simulink model "submarine"  (Simulink 6.3)
settings: Solver=ode45  StartTime=0.0  StopTime=15.0  RelTol=1e-3
settings Model: LastModifiedBy=Yuantao Gu

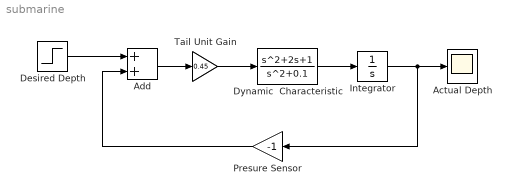
== system submarine ==
  Actual Depth : Scope
      settings: TimeRange=15  YMin=-120  YMax=0
  Add : Sum  OutScaling=2^-10
  Desired Depth : Step  Time=0  After=-60  SampleTime=0
  Dynamic  Characteristic : TransferFcn  Numerator=[1 2 1]  Denominator=[1 0 0.1]
  Integrator : Integrator
  Presure Sensor : Gain  Orientation=left  Gain=-1
  Tail Unit Gain : Gain  Gain=0.45
  wires:
  Desired Depth/1 -> Add/1
  Add/1 -> Tail Unit Gain/1
  Tail Unit Gain/1 -> Dynamic  Characteristic/1
  Dynamic  Characteristic/1 -> Integrator/1
  Presure Sensor/1 -> Add/2
  Integrator/1 -> Presure Sensor/1, Actual Depth/1
